simulink model "Copy_of_manipulator2c12pid"  (Simulink 10.0)
settings: Solver=FixedStepAuto  StartTime=0.0  StopTime=10.2557  FixedStep=0.001  RelTol=1e-3
libraries: simulink x1
settings Model: Creator=dell  LastModifiedBy=JOHN WICK
settings DataIOCC: SaveFormat=Dataset
settings OptimizationCC: LifeSpan=auto
settings DebuggingCC: UnderspecifiedInitializationDetection=Simplified  MergeDetectMultiDrivingBlocksExec=error  SFUnexpectedBacktrackingDiag=error  SFNoUnconditionalDefaultTransitionDiag=error  SFExecutionAtInitializationDiag=warning
settings HardwareCC: ProdBitPerPointer=64  ProdBitPerSizeT=64  ProdBitPerPtrDiffT=64  ProdLargestAtomicFloat=Float  ProdIntDivRoundTo=Zero  ProdEndianess=LittleEndian  ProdWordSize=64  ProdHWDeviceType=Intel->x86-64 (Windows64)
settings ModelReferenceCC: PropagateSignalLabelsOutOfModel=on
settings GRTTargetCC: TargetLangStandard=C99 (ISO)  CombineOutputUpdateFcns=on  GRTInterface=off
settings ConfigComp: CovMetricSettings=dwe  CovHtmlReporting=off  CovSaveCumulativeToWorkspaceVar=off  CovSaveSingleToWorkspaceVar=off

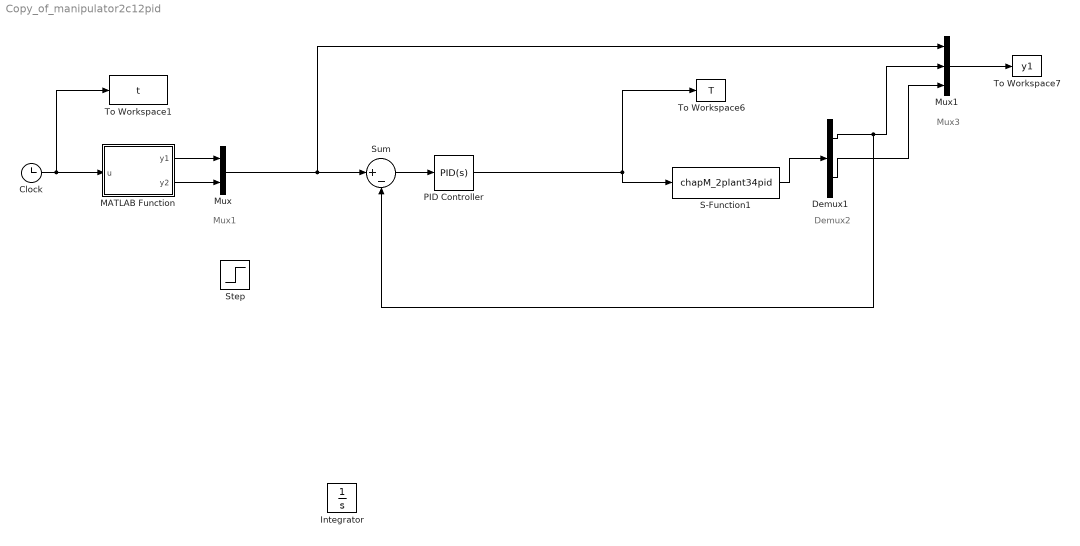
== system Copy_of_manipulator2c12pid ==
  note: Demux2
  note: Mux3
  note: Mux1
  Clock : Clock
  Demux1 : Demux  Outputs=2
  Integrator : Integrator
  MATLAB Function : MATLAB Function  TreatAsAtomicUnit=on
  Mux : Mux  Inputs=2
  Mux1 : Mux  Inputs=3
  PID Controller : simulink/Continuous/PID Controller  Controller=PID  Form=Parallel  TimeDomain=Continuous-time  SampleTime=-1  IntegratorMethod=Forward Euler  FilterMethod=Forward Euler  ControllerParametersSource=internal  P=5000  I=500  D=2000  UseFilter=on  N=100  TunerSelectOption=Transfer Function Based (PID Tuner App)  InitialConditionSource=internal  InitialConditionForIntegrator=0  InitialConditionForFilter=0  DifferentiatorICPrevScaledInput=0  ExternalReset=none  TrackingMode=off  Kt=1  LimitOutput=off  UpperSaturationLimit=inf  LowerSaturationLimit=-inf  LinearizeAsGain=on  AntiWindupMode=none  Kb=1  POutMin=[]  POutMax=[]  IOutMin=[]  IOutMax=[]  DOutMin=[]  DOutMax=[]  NOutMin=[]  NOutMax=[]  SumOutMin=[]  SumOutMax=[]  SaturationOutMin=[]  SaturationOutMax=[]  PParamMin=[]  PParamMax=[]  IParamMin=[]  IParamMax=[]  DParamMin=[]  DParamMax=[]  NParamMin=[]  NParamMax=[]  KbParamMin=[]  KbParamMax=[]  KtParamMin=[]  KtParamMax=[]  KbOutMin=[]  KbOutMax=[]  KtOutMin=[]  KtOutMax=[]  IntegratorOutMin=[]  IntegratorOutMax=[]  FilterOutMin=[]  FilterOutMax=[]  SumI1OutMin=[]  SumI1OutMax=[]  SumI2OutMin=[]  SumI2OutMax=[]  SumI3OutMin=[]  SumI3OutMax=[]  SumI4OutMin=[]  SumI4OutMax=[]  SumDOutMin=[]  SumDOutMax=[]  DifferentiatorOutMin=[]  DifferentiatorOutMax=[]  FilterDiffOutCoefMin=[]  FilterDiffOutCoefMax=[]  ReciprocalOutMin=[]  ReciprocalOutMax=[]  SumDenOutMin=[]  SumDenOutMax=[]  SumNumOutMin=[]  SumNumOutMax=[]  DivideOutMin=[]  DivideOutMax=[]  IntegratorContinuousStateAttributes=''  IntegratorStateMustResolveToSignalObject=off  IntegratorRTWStateStorageClass=Auto  FilterContinuousStateAttributes=''  FilterStateMustResolveToSignalObject=off  FilterRTWStateStorageClass=Auto  ParallelPVariant=InternalParameters  IdealPVariant=Disabled  IVariant=InternalParameters  DVariant=InternalParameters  IntegratorVariant=Continuous  SatVariant=Disabled  AWVariant=Passthrough  PCopyVariant=Disabled  TRVariant=Disabled  FdbkBlocksVariant=Forward  IdealPFdbkVariant=Disabled  SatFdbkVariant=Disabled  DerivativeFilterVariant=ContFilter  NVariant=InternalParameters  NCopyVariant=Disabled  FilterICVariant=InternalICsFilter  IntegratorICVariant=InternalICs  ExternalResetVariant=Disabled  TRSumVariant=Passthrough  SumFdbkVariant=Disabled  SumVariant=Sum_PID
  S-Function1 : S-Function  FunctionName=chapM_2plant34pid  SFunctionDeploymentMode=off  EnableBusSupport=off
  Step : Step  Time=0  SampleTime=0
  Sum : Sum  Inputs=|+-
  To Workspace1 : ToWorkspace  VariableName=t  SampleTime=-1
  To Workspace6 : ToWorkspace  VariableName=T  SampleTime=-1
  To Workspace7 : ToWorkspace  VariableName=y1  SampleTime=-1
  wires:
  MATLAB Function/2(y2) -> Mux/2
  MATLAB Function/1(y1) -> Mux/1
  PID Controller/1 -> S-Function1/1, To Workspace6/1
  S-Function1/1 -> Demux1/1
  Clock/1 -> To Workspace1/1, MATLAB Function/1(u)
  Mux1/1 -> To Workspace7/1
  Demux1/1 -> Mux1/2, Sum/2
  Demux1/2 -> Mux1/3
  Sum/1 -> PID Controller/1
  Mux/1 -> Mux1/1, Sum/1

== matlab function MATLAB Function ==
  data: u input double; y1 output double; y2 output double
function [y1,y2]=fcn(u)
tnode=[0	2.380632392	3.505666959	4.275059855	6.612705584	7.88863381	10.25572392];

curve1=[0.001998939	-0.00969027	-6.76E-17	0	-0.34906585
-0.001673717	0.025282709	-0.12488671	0.198206232	-0.467029894
-0.000231492	0.005058859	-0.018539585	-0.050338837	-0.249200835
-0.002885392	0.050441185	-0.309557826	0.779074762	-1.13564903
0.014699294	-0.41468823	4.304087995	-19.56004623	32.48850571
-0.009354817	0.344328089	-4.677314702	27.67395176	-60.66442266];

curve2=[-0.003220844	0.015607104	6.76E-17	0	0.34906585
0.007050914	-0.082206011	0.349285605	-0.554347084	0.678990006
-0.011627037	0.179708689	-1.027992961	2.664506224	-2.142066916
0.004386156	-0.094120744	0.727962863	-2.340037942	3.206614549
-0.008472244	0.2459945	-2.645660091	12.53247896	-21.38027934
0.003219462	-0.122931833	1.719827019	-10.42600718	23.89749316];

if u>=tnode(1)&&u<tnode(2)
    y1=curve1(1,:)*[u^4,u^3,u^2,u,1]';
    y2=curve2(1,:)*[u^4,u^3,u^2,u,1]';
elseif u>=tnode(2)&&u<tnode(3)
    y1=curve1(2,:)*[u^4,u^3,u^2,u,1]';
    y2=curve2(2,:)*[u^4,u^3,u^2,u,1]';
elseif u>=tnode(3)&&u<tnode(4)
    y1=curve1(3,:)*[u^4,u^3,u^2,u,1]';
    y2=curve2(3,:)*[u^4,u^3,u^2,u,1]';
elseif u>=tnode(4)&&u<tnode(5)
    y1=curve1(4,:)*[u^4,u^3,u^2,u,1]';
    y2=curve2(4,:)*[u^4,u^3,u^2,u,1]';
elseif u>=tnode(5)&&u<tnode(6)
    y1=curve1(5,:)*[u^4,u^3,u^2,u,1]';
    y2=curve2(5,:)*[u^4,u^3,u^2,u,1]';
else u>=tnode(6)&&u<=tnode(7)
    y1=curve1(6,:)*[u^4,u^3,u^2,u,1]';
    y2=curve2(6,:)*[u^4,u^3,u^2,u,1]';
end
